simulink model "sampleModel1686"  (R2023a)
settings: Solver=VariableStepAuto  StartTime=0.0  StopTime=10.0  RelTol=1e-3
libraries: hdlsllib x4, simulink x3
settings Model: Creator=user1  LastModifiedBy=user1

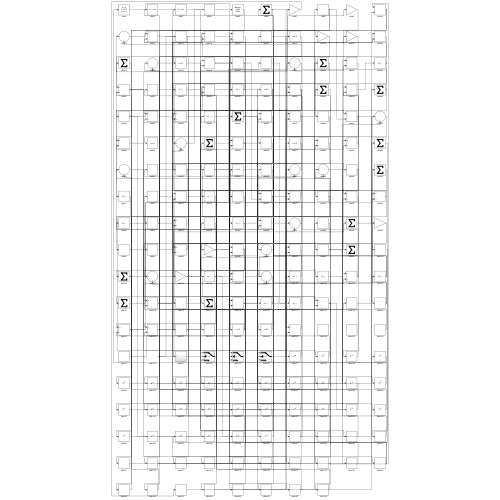
[thumbnail: Simulink's stored preview of the top-level diagram]
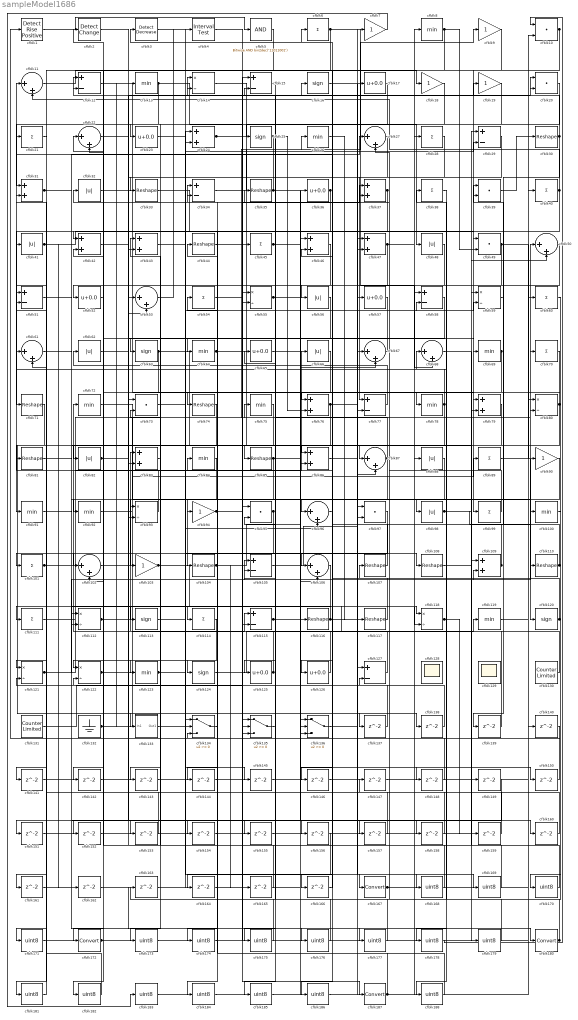
== system sampleModel1686 ==
  cfblk1 : hdlsllib/Logic and Bit Operations/Detect Rise Positive  vinit=0  OutDataTypeStr=boolean
  cfblk{10,20,39,49,73,95,97} (7 alike) : DotProduct  OutDataTypeStr=Inherit: Inherit via internal rule
  cfblk{8,13,26,64,69,72,75,78,84,91..92,100,119,123} (14 alike) : MinMax
  cfblk{6,21,28,38,40,45,54,60,70,89,99,101,111,114} (14 alike) : Sum  Inputs=+
  cfblk{11,22,27,50,53,61,67..68,87,96,102,106} (12 alike) : Sum  Inputs=|++
  cfblk{7,9,18..19,90,94,103} (7 alike) : Gain
  cfblk{30,33,35,44,71,74,81,85,104,107..108,110,116..117} (14 alike) : Reshape
  cfblk{12,15,29,34,51,58,77,105,115,127} (10 alike) : Sum  Inputs=+-
  cfblk{24,31,37,42..43,46..47,76,79,83,86,109} (12 alike) : Sum
  cfblk{14,55,59,80,93,112,118,121..122} (9 alike) : Product  Inputs=*/  RndMeth=Zero  SaturateOnIntegerOverflow=on
  cfblk{16,25,63,113,120,124} (6 alike) : Signum
  cfblk{17,23,36,52,57,65,125..126} (8 alike) : Bias  Bias=0.0  SaturateOnIntegerOverflow=off
  cfblk128 : Scope
      settings: Floating=on
  cfblk129 : Scope
      settings: Floating=on
  cfblk130 : hdlsllib/Sources/Counter Limited  uplimit=7  tsamp=-1
  cfblk131 : hdlsllib/Sources/Counter Limited  uplimit=7  tsamp=-1
  cfblk132 : Ground
  cfblk133 : Subsystem
      settings: LibrarySourceBlock=|
      | hdlsllib/Ports &
      | Subsystems/Subsystem
  cfblk134 : Switch  SaturateOnIntegerOverflow=off  InputSameDT=off
  cfblk135 : Switch  SaturateOnIntegerOverflow=off  InputSameDT=off
  cfblk136 : Switch  SaturateOnIntegerOverflow=off  InputSameDT=off
  cfblk{137..166} (30 alike) : Delay  SampleTime=1
  cfblk{167,172,180,187} (4 alike) : DataTypeConversion  SaturateOnIntegerOverflow=off  RndMeth=Floor
  cfblk{168..171,173..179,181..186,188} (18 alike) : DataTypeConversion  OutDataTypeStr=uint8  SaturateOnIntegerOverflow=off  RndMeth=Floor
  cfblk2 : simulink/Logic and Bit Operations/Detect Change  vinit=0  OutDataTypeStr=boolean
      settings: LibrarySourceBlock=|
      | hdlsllib/Logic and Bit
      | Operations/Detect
      | Change
  cfblk3 : simulink/Logic and Bit Operations/Detect Decrease  vinit=0.0  OutDataTypeStr=boolean
      settings: LibrarySourceBlock=|
      | hdlsllib/Logic and Bit
      | Operations/Detect
      | Decrease
  cfblk{32,41,48,56,62,66,82,88,98} (9 alike) : Abs  SaturateOnIntegerOverflow=off
  cfblk4 : hdlsllib/Logic and Bit Operations/Interval Test  IntervalClosedRight=on  uplimit=0.5  IntervalClosedLeft=on  lowlimit=-0.5  OutDataTypeStr=boolean
  cfblk5 : simulink/Logic and Bit Operations/Bitwise Operator  logicop=AND  UseBitMask=on  BitMask=bin2dec('11011001')  BitMaskRealWorld=Stored Integer
      settings: LibrarySourceBlock=|
      | hdlsllib/Logic and Bit
      | Operations/Bitwise
      | Operator
  wires:
  cfblk97/1 -> cfblk172/1
  cfblk35/1 -> cfblk33/1, cfblk148/1
  cfblk9/1 -> cfblk99/1
  cfblk27/1 -> cfblk77/1
  cfblk132/1 -> cfblk115/1, cfblk13/1
  cfblk24/1 -> cfblk48/1, cfblk106/1
  cfblk26/1 -> cfblk117/1
  cfblk121/1 -> cfblk26/1, cfblk105/1
  cfblk103/1 -> cfblk119/1, cfblk96/2
  cfblk63/1 -> cfblk85/1, cfblk83/2
  cfblk98/1 -> cfblk50/1, cfblk50/2
  cfblk39/1 -> cfblk30/1
  cfblk71/1 -> cfblk133/1(In1)
  cfblk53/1 -> cfblk4/1
  cfblk44/1 -> cfblk135/1
  cfblk84/1 -> cfblk104/1
  cfblk92/1 -> cfblk98/1
  cfblk73/1 -> cfblk167/1
  cfblk118/1 -> cfblk159/1, cfblk188/1
  cfblk120/1 -> cfblk70/1, cfblk27/2
  cfblk86/1 -> cfblk127/1
  cfblk93/1 -> cfblk11/1
  cfblk36/1 -> cfblk71/1, cfblk143/1
  cfblk79/1 -> cfblk114/1
  cfblk124/1 -> cfblk8/1
  cfblk5/1 -> cfblk51/1
  cfblk77/1 -> cfblk62/1
  cfblk32/1 -> cfblk115/2
  cfblk117/1 -> cfblk16/1
  cfblk12/1 -> cfblk79/1
  cfblk30/1 -> cfblk2/1, cfblk139/1
  cfblk1/1 -> cfblk5/1
  cfblk56/1 -> cfblk63/1
  cfblk126/1 -> cfblk72/1
  cfblk14/1 -> cfblk87/1
  cfblk48/1 -> cfblk52/1
  cfblk66/1 -> cfblk124/1
  cfblk72/1 -> cfblk96/1
  cfblk65/1 -> cfblk116/1
  cfblk46/1 -> cfblk56/1
  cfblk122/1 -> cfblk24/2, cfblk110/1
  cfblk54/1 -> cfblk187/1
  cfblk62/1 -> cfblk69/1
  cfblk45/1 -> cfblk118/1, cfblk157/1
  cfblk96/1 -> cfblk46/2
  cfblk136/1 -> cfblk57/1
  cfblk116/1 -> cfblk111/1, cfblk58/2
  cfblk67/1 -> cfblk64/1
  cfblk94/1 -> cfblk25/1, cfblk20/2
  cfblk76/1 -> cfblk150/1, cfblk151/1
  cfblk130/1 -> cfblk83/1
  cfblk112/1 -> cfblk45/1, cfblk20/1, cfblk160/1
  cfblk57/1 -> cfblk113/1
  cfblk33/1 -> cfblk77/2
  cfblk34/1 -> cfblk9/1
  cfblk85/1 -> cfblk123/1, cfblk67/2
  cfblk6/1 -> cfblk68/2, cfblk93/2
  cfblk99/1 -> cfblk32/1
  cfblk80/1 -> cfblk91/1, cfblk78/1
  cfblk41/1 -> cfblk49/1, cfblk162/1
  cfblk55/1 -> cfblk125/1, cfblk100/1
  cfblk134/1 -> cfblk84/1
  cfblk111/1 -> cfblk58/1
  cfblk50/1 -> cfblk82/1
  cfblk74/1 -> cfblk101/1
  cfblk102/1 -> cfblk89/1
  cfblk83/1 -> cfblk43/1
  cfblk110/1 -> cfblk3/1, cfblk39/2
  cfblk101/1 -> cfblk66/1, cfblk161/1
  cfblk119/1 -> cfblk40/1
  cfblk47/1 -> cfblk19/1, cfblk166/1
  cfblk95/1 -> cfblk121/1, cfblk164/1
  cfblk69/1 -> cfblk94/1, cfblk154/1
  cfblk114/1 -> cfblk122/1
  cfblk19/1 -> cfblk23/1
  cfblk109/1 -> cfblk6/1, cfblk81/1
  cfblk59/1 -> cfblk39/1
  cfblk64/1 -> cfblk109/1, cfblk37/1
  cfblk61/1 -> cfblk180/1
  cfblk10/1 -> cfblk102/1, cfblk146/1
  cfblk42/1 -> cfblk14/1
  cfblk123/1 -> cfblk75/1, cfblk145/1
  cfblk105/1 -> cfblk17/1
  cfblk88/1 -> cfblk103/1
  cfblk87/1 -> cfblk65/1, cfblk153/1
  cfblk11/1 -> cfblk18/1
  cfblk40/1 -> cfblk11/2, cfblk186/1
  cfblk20/1 -> cfblk42/1
  cfblk31/1 -> cfblk112/1, cfblk118/2, cfblk27/1
  cfblk90/1 -> cfblk112/2
  cfblk37/1 -> cfblk92/1, cfblk74/1, cfblk41/1
  cfblk127/1 -> cfblk12/1
  cfblk131/1 -> cfblk55/1
  cfblk82/1 -> cfblk42/2, cfblk14/2
  cfblk115/1 -> cfblk109/2, cfblk158/1
  cfblk104/1 -> cfblk80/2, cfblk165/1
  cfblk25/1 -> cfblk43/2, cfblk76/2
  cfblk135/1 -> cfblk95/2
  cfblk89/1 -> cfblk120/1
  cfblk78/1 -> cfblk136/3, cfblk126/1, cfblk31/2
  cfblk52/1 -> cfblk22/1
  cfblk23/1 -> cfblk134/1
  cfblk113/1 -> cfblk59/2
  cfblk51/1 -> cfblk86/1
  cfblk8/1 -> cfblk49/2, cfblk156/1, cfblk171/1
  cfblk43/1 -> cfblk108/1
  cfblk29/1 -> cfblk93/1
  cfblk133/1(Out1) -> cfblk29/2
  cfblk49/1 -> cfblk90/1, cfblk76/1
  cfblk13/1 -> cfblk31/1, cfblk135/3
  cfblk125/1 -> cfblk22/2, cfblk34/1
  cfblk107/1 -> cfblk21/1
  cfblk2/1 -> cfblk53/1
  cfblk22/1 -> cfblk137/1
  cfblk137/1 -> cfblk51/2
  cfblk91/1 -> cfblk138/1
  cfblk138/1 -> cfblk127/2
  cfblk139/1 -> cfblk24/1
  cfblk140/1 -> cfblk1/1
  cfblk21/1 -> cfblk141/1
  cfblk141/1 -> cfblk136/2
  cfblk18/1 -> cfblk142/1
  cfblk142/1 -> cfblk135/2
  cfblk143/1 -> cfblk47/2
  cfblk75/1 -> cfblk144/1
  cfblk144/1 -> cfblk80/1
  cfblk145/1 -> cfblk105/2
  cfblk146/1 -> cfblk67/1
  cfblk147/1 -> cfblk79/2
  cfblk148/1 -> cfblk95/1
  cfblk108/1 -> cfblk149/1
  cfblk150/1 -> cfblk68/1
  cfblk151/1 -> cfblk53/2
  cfblk58/1 -> cfblk152/1
  cfblk152/1 -> cfblk87/2
  cfblk153/1 -> cfblk102/2
  cfblk154/1 -> cfblk106/2
  cfblk81/1 -> cfblk155/1
  cfblk155/1 -> cfblk59/1
  cfblk157/1 -> cfblk46/1
  cfblk158/1 -> cfblk121/2
  cfblk159/1 -> cfblk122/2
  cfblk160/1 -> cfblk37/2
  cfblk161/1 -> cfblk134/2
  cfblk100/1 -> cfblk163/1
  cfblk163/1 -> cfblk136/1
  cfblk164/1 -> cfblk134/3
  cfblk165/1 -> cfblk12/2
  cfblk166/1 -> cfblk86/2
  cfblk167/1 -> cfblk140/1, cfblk107/1
  cfblk3/1 -> cfblk168/1
  cfblk168/1 -> cfblk73/1
  cfblk16/1 -> cfblk169/1
  cfblk169/1 -> cfblk73/2
  cfblk60/1 -> cfblk170/1
  cfblk170/1 -> cfblk29/1
  cfblk171/1 -> cfblk60/1
  cfblk172/1 -> cfblk55/2, cfblk88/1
  cfblk17/1 -> cfblk173/1
  cfblk173/1 -> cfblk97/1
  cfblk156/1 -> cfblk174/1
  cfblk174/1 -> cfblk97/2
  cfblk15/1 -> cfblk175/1
  cfblk175/1 -> cfblk44/1
  cfblk4/1 -> cfblk176/1
  cfblk176/1 -> cfblk15/1
  cfblk162/1 -> cfblk177/1
  cfblk177/1 -> cfblk15/2
  cfblk38/1 -> cfblk178/1
  cfblk178/1 -> cfblk10/1
  cfblk68/1 -> cfblk179/1
  cfblk179/1 -> cfblk38/1
  cfblk180/1 -> cfblk147/1, cfblk35/1
  cfblk149/1 -> cfblk181/1
  cfblk181/1 -> cfblk61/1
  cfblk70/1 -> cfblk182/1
  cfblk182/1 -> cfblk61/2
  cfblk7/1 -> cfblk183/1
  cfblk183/1 -> cfblk47/1
  cfblk106/1 -> cfblk184/1
  cfblk184/1 -> cfblk7/1
  cfblk28/1 -> cfblk185/1
  cfblk185/1 -> cfblk36/1
  cfblk186/1 -> cfblk28/1
  cfblk187/1 -> cfblk34/2, cfblk10/2
  cfblk188/1 -> cfblk54/1

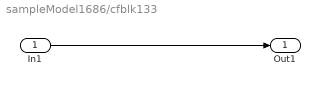
== system sampleModel1686/cfblk133 ==
  In1 : Inport
  Out1 : Outport
  wires:
  In1/1 -> Out1/1
